simulink model "Simulacao_Modelos"  (R2015a)
settings: Solver=ode45  StartTime=0.0  StopTime=1430  RelTol=1e-3
settings Model: Creator=gabri  LastModifiedBy=gabri

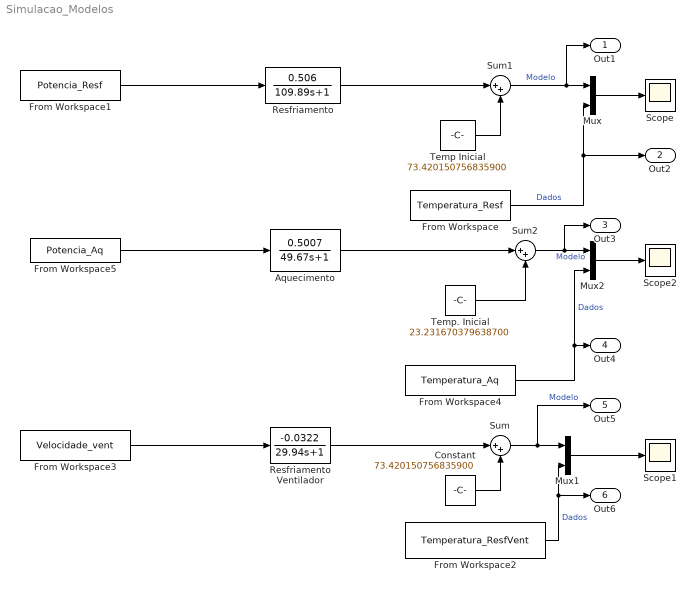
== system Simulacao_Modelos ==
  Aquecimento : TransferFcn  Numerator=[0.5007]  Denominator=[49.67 1]
  Constant : Constant  Value=73.420150756835900
  From Workspace : FromWorkspace  VariableName=Temperatura_Resf  SampleTime=0
  From Workspace1 : FromWorkspace  VariableName=Potencia_Resf  SampleTime=0
  From Workspace2 : FromWorkspace  VariableName=Temperatura_ResfVent  SampleTime=0
  From Workspace3 : FromWorkspace  VariableName=Velocidade_vent  SampleTime=0
  From Workspace4 : FromWorkspace  VariableName=Temperatura_Aq  SampleTime=0
  From Workspace5 : FromWorkspace  VariableName=Potencia_Aq  SampleTime=0
  Mux : Mux  Inputs=2
  Mux1 : Mux  Inputs=2
  Mux2 : Mux  Inputs=2
  Resfriamento : TransferFcn  Numerator=[0.506]  Denominator=[109.89 1]
  Resfriamento Ventilador : TransferFcn  Numerator=[-0.0322]  Denominator=[29.94 1]
  Scope : Scope
      settings: ShowLegends=on
  Scope1 : Scope
      settings: ShowLegends=on
  Scope2 : Scope
      settings: ShowLegends=on  SaveName=ScopeData2
  Sum : Sum  Inputs=|++
  Sum1 : Sum  Inputs=|++
  Sum2 : Sum  Inputs=|++
  Temp Inicial : Constant  Value=73.420150756835900
  Temp. Inicial : Constant  Value=23.231670379638700
  Out1 : Outport
  Out2 : Outport  Port=2
  Out3 : Outport  Port=3
  Out4 : Outport  Port=4
  Out5 : Outport  Port=5
  Out6 : Outport  Port=6
  wires:
  Mux/1 -> Scope/1
  From Workspace1/1 -> Resfriamento/1
  From Workspace3/1 -> Resfriamento Ventilador/1
  Mux2/1 -> Scope2/1
  From Workspace5/1 -> Aquecimento/1
  Resfriamento Ventilador/1 -> Sum/1
  Constant/1 -> Sum/2
  Mux1/1 -> Scope1/1
  From Workspace2/1 -> Out6/1, Mux1/2  "Dados"
  Sum1/1 -> Out1/1, Mux/1  "Modelo"
  From Workspace/1 -> Mux/2, Out2/1  "Dados"
  Sum2/1 -> Out3/1, Mux2/1  "Modelo"
  From Workspace4/1 -> Mux2/2, Out4/1  "Dados"
  Temp. Inicial/1 -> Sum2/2
  Sum/1 -> Out5/1, Mux1/1  "Modelo"
  Aquecimento/1 -> Sum2/1
  Resfriamento/1 -> Sum1/1
  Temp Inicial/1 -> Sum1/2
